simulink model "Sim"  (R2021b)
settings: Solver=VariableStepAuto  StartTime=0.0  StopTime=10.0  RelTol=1e-3
libraries: cstblocks x1
settings Model: Creator=saigon  LastModifiedBy=saigon

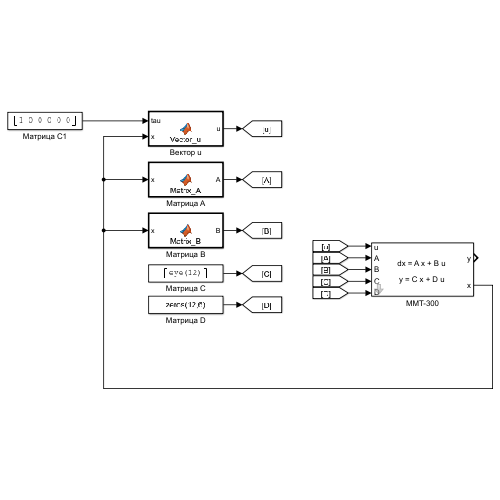
[thumbnail: Simulink's stored preview of the top-level diagram]
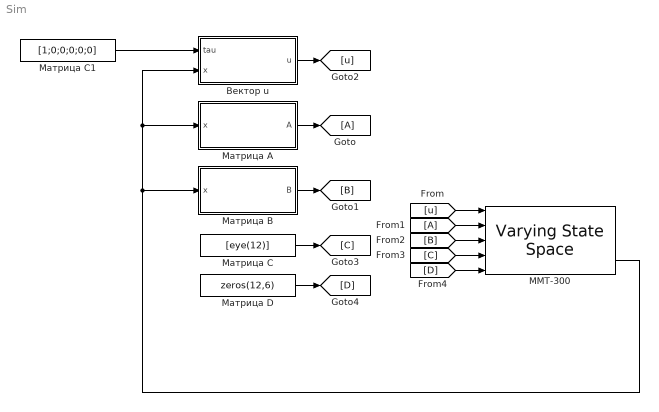
== system Sim ==
  MMT-300 : cstblocks/Linear Parameter Varying/Varying State Space  x0=zeros(12,1)  xNames=''  OutputX=on  OutputDX=off
  Вектор u : MATLAB Function  TreatAsAtomicUnit=on
  Матрица A : MATLAB Function  TreatAsAtomicUnit=on
  Матрица B : MATLAB Function  TreatAsAtomicUnit=on
  Матрица C : Constant  Value=[eye(12)]
  Матрица C1 : Constant  Value=[1;0;0;0;0;0]
  Матрица D : Constant  Value=zeros(12,6)
  wires:
  [C] -> MMT-300/4
  [D] -> MMT-300/5
  Вектор u/1(u) -> [u]
  [B] -> MMT-300/3
  Матрица C/1 -> [C]
  Матрица B/1(B) -> [B]
  Матрица D/1 -> [D]
  [u] -> MMT-300/1
  [A] -> MMT-300/2
  Матрица A/1(A) -> [A]
  Матрица C1/1 -> Вектор u/1(tau)
  MMT-300/2 -> Матрица B/1(x), Матрица A/1(x), Вектор u/2(x)

== matlab function Sim/Матрица A ==
  data: x input size=12; A output size=[12 12]; MMT300 parameter
function A = Matrix_A(x, MMT300)
n = 6;
eta = x(1:n); 
v = x(7:end);
J = MMT300.J(eta);
M = MMT300.M;
C = MMT300.C(MMT300,v);

A = [ zeros(n), J^-1;
      zeros(n), -M^-1 * ( C(v) ) ];

== matlab function Sim/Матрица B ==
  data: x input size=12; B output size=[12 6]; MMT300 parameter
function B = Matrix_B(x, MMT300)
n = 6;
B = [zeros(n); MMT300.M^-1];

== matlab function Sim/Вектор u ==
  data: tau input [-127..127]; x input size=12; u output size=6; MMT300 parameter
function u = Vector_u(tau, x, MMT300)
n = 6;
eta = x(1:n); 

u = -MMT300.g(MMT300,eta) + tau;
